simulink model "course_hold"  (Simulink 7.7)
settings: Solver=ode3  StartTime=0.0  StopTime=10.0  RelTol=1e-3
undefined symbols (not defined in the file): g, k_i_chi, k_p_chi, V_g
settings Model: Creator=prattmic  LastModifiedBy=prattmic
settings OptimizationCC: InlineParams=on
settings HardwareCC: ProdLargestAtomicInteger=Long  ProdLargestAtomicFloat=Double  ProdEndianess=LittleEndian  ProdHWDeviceType=ARM Compatible->ARM Cortex

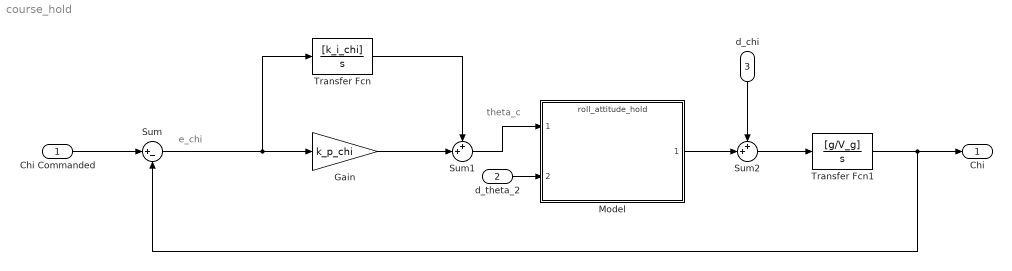
== system course_hold ==
  note: e_chi
  note: theta_c
  Chi Commanded : Inport
  d_theta_2 : Inport  Port=2
  d_chi : Inport  Port=3
  Gain : Gain  Gain=k_p_chi
  Model : ModelReference  ModelNameDialog=roll_attitude_hold  SimulationMode=Normal  ModelReferenceVersion=1.13  CopyOfModelName=roll_attitude_hold  DefaultDataLogging=on
  Sum : Sum  Inputs=|+-
  Sum1 : Sum  Inputs=++|
  Sum2 : Sum  Inputs=++|
  Transfer Fcn : TransferFcn  Numerator=[k_i_chi]  Denominator=[1 0]
  Transfer Fcn1 : TransferFcn  Numerator=[g/V_g]  Denominator=[1 0]
  Chi : Outport
  wires:
  Chi Commanded/1 -> Sum/1
  Sum/1 -> Gain/1, Transfer Fcn/1
  Sum2/1 -> Transfer Fcn1/1
  Transfer Fcn1/1 -> Chi/1, Sum/2
  Transfer Fcn/1 -> Sum1/1
  Gain/1 -> Sum1/2
  d_chi/1 -> Sum2/1
  Sum1/1 -> Model/1
  Model/1 -> Sum2/2
  d_theta_2/1 -> Model/2
